simulink library "MIL_Test"  (Simulink 7.0)
values from neighbouring files (symbols this model uses):
  TID = min('TI' == AFT(1:2))    [PAS_callback.m]    (also in PSTID_callback.m = [block '/TID'])
undefined symbols (not defined in the file or in its folder): getdatatypespecs, slcm, StepSize
libraries: simulink x71, MIL_Test x6
(part 6 of 11)

== system MIL_Test/Test Data/Feature generation/Generate timed limited increase/Subsystem/Subsystem39 ==
  In1 : Inport  OutDataType=sfix(16)  OutScaling=2^0
  In2 : Inport  Port=2  OutDataType=sfix(16)  OutScaling=2^0
  In3 : Inport  Port=3  OutDataType=sfix(16)  OutScaling=2^0
  Output1 : Sum  Inputs=|+-+  OutDataType=sfix(16)  OutScaling=2^0  SaturateOnIntegerOverflow=on  InputSameDT=on
  RO : RelationalOperator  Operator=>  LogicOutDataTypeMode=boolean
  Switch : Switch  Criteria=u2 > Threshold
  Out1 : Outport  OutDataType=sfix(16)  OutScaling=2^0
  wires:
  In3/1 -> Output1/3
  Output1/1 -> Switch/1
  RO/1 -> Switch/2
  Switch/1 -> Out1/1
  In2/1 -> RO/1, Output1/1, Switch/3  "U(k)"
  In1/1 -> RO/2, Output1/2

== system MIL_Test/Test Data/Feature generation/Generate timed limited increase/Subsystem/Subsystem4 ==
  In1 : Inport  OutDataType=sfix(16)  OutScaling=2^0
  In2 : Inport  Port=2  OutDataType=sfix(16)  OutScaling=2^0
  In3 : Inport  Port=3  OutDataType=sfix(16)  OutScaling=2^0
  Output1 : Sum  Inputs=|+-+  OutDataType=sfix(16)  OutScaling=2^0  SaturateOnIntegerOverflow=on  InputSameDT=on
  RO : RelationalOperator  Operator=>  LogicOutDataTypeMode=boolean
  Switch : Switch  Criteria=u2 > Threshold
  Out1 : Outport  OutDataType=sfix(16)  OutScaling=2^0
  wires:
  In3/1 -> Output1/3
  Output1/1 -> Switch/1
  RO/1 -> Switch/2
  Switch/1 -> Out1/1
  In2/1 -> RO/1, Output1/1, Switch/3  "U(k)"
  In1/1 -> RO/2, Output1/2

== system MIL_Test/Test Data/Feature generation/Generate timed limited increase/Subsystem/Subsystem40 ==
  In1 : Inport  OutDataType=sfix(16)  OutScaling=2^0
  In2 : Inport  Port=2  OutDataType=sfix(16)  OutScaling=2^0
  In3 : Inport  Port=3  OutDataType=sfix(16)  OutScaling=2^0
  Output1 : Sum  Inputs=|+-+  OutDataType=sfix(16)  OutScaling=2^0  SaturateOnIntegerOverflow=on  InputSameDT=on
  RO : RelationalOperator  Operator=>  LogicOutDataTypeMode=boolean
  Switch : Switch  Criteria=u2 > Threshold
  Out1 : Outport  OutDataType=sfix(16)  OutScaling=2^0
  wires:
  In3/1 -> Output1/3
  Output1/1 -> Switch/1
  RO/1 -> Switch/2
  Switch/1 -> Out1/1
  In2/1 -> RO/1, Output1/1, Switch/3  "U(k)"
  In1/1 -> RO/2, Output1/2

== system MIL_Test/Test Data/Feature generation/Generate timed limited increase/Subsystem/Subsystem41 ==
  In1 : Inport  OutDataType=sfix(16)  OutScaling=2^0
  In2 : Inport  Port=2  OutDataType=sfix(16)  OutScaling=2^0
  In3 : Inport  Port=3  OutDataType=sfix(16)  OutScaling=2^0
  Output1 : Sum  Inputs=|+-+  OutDataType=sfix(16)  OutScaling=2^0  SaturateOnIntegerOverflow=on  InputSameDT=on
  RO : RelationalOperator  Operator=>  LogicOutDataTypeMode=boolean
  Switch : Switch  Criteria=u2 > Threshold
  Out1 : Outport  OutDataType=sfix(16)  OutScaling=2^0
  wires:
  In3/1 -> Output1/3
  Output1/1 -> Switch/1
  RO/1 -> Switch/2
  Switch/1 -> Out1/1
  In2/1 -> RO/1, Output1/1, Switch/3  "U(k)"
  In1/1 -> RO/2, Output1/2

== system MIL_Test/Test Data/Feature generation/Generate timed limited increase/Subsystem/Subsystem42 ==
  In1 : Inport  OutDataType=sfix(16)  OutScaling=2^0
  In2 : Inport  Port=2  OutDataType=sfix(16)  OutScaling=2^0
  In3 : Inport  Port=3  OutDataType=sfix(16)  OutScaling=2^0
  Output1 : Sum  Inputs=|+-+  OutDataType=sfix(16)  OutScaling=2^0  SaturateOnIntegerOverflow=on  InputSameDT=on
  RO : RelationalOperator  Operator=>  LogicOutDataTypeMode=boolean
  Switch : Switch  Criteria=u2 > Threshold
  Out1 : Outport  OutDataType=sfix(16)  OutScaling=2^0
  wires:
  In3/1 -> Output1/3
  Output1/1 -> Switch/1
  RO/1 -> Switch/2
  Switch/1 -> Out1/1
  In2/1 -> RO/1, Output1/1, Switch/3  "U(k)"
  In1/1 -> RO/2, Output1/2

== system MIL_Test/Test Data/Feature generation/Generate timed limited increase/Subsystem/Subsystem43 ==
  In1 : Inport  OutDataType=sfix(16)  OutScaling=2^0
  In2 : Inport  Port=2  OutDataType=sfix(16)  OutScaling=2^0
  In3 : Inport  Port=3  OutDataType=sfix(16)  OutScaling=2^0
  Output1 : Sum  Inputs=|+-+  OutDataType=sfix(16)  OutScaling=2^0  SaturateOnIntegerOverflow=on  InputSameDT=on
  RO : RelationalOperator  Operator=>  LogicOutDataTypeMode=boolean
  Switch : Switch  Criteria=u2 > Threshold
  Out1 : Outport  OutDataType=sfix(16)  OutScaling=2^0
  wires:
  In3/1 -> Output1/3
  Output1/1 -> Switch/1
  RO/1 -> Switch/2
  Switch/1 -> Out1/1
  In2/1 -> RO/1, Output1/1, Switch/3  "U(k)"
  In1/1 -> RO/2, Output1/2

== system MIL_Test/Test Data/Feature generation/Generate timed limited increase/Subsystem/Subsystem44 ==
  In1 : Inport  OutDataType=sfix(16)  OutScaling=2^0
  In2 : Inport  Port=2  OutDataType=sfix(16)  OutScaling=2^0
  In3 : Inport  Port=3  OutDataType=sfix(16)  OutScaling=2^0
  Output1 : Sum  Inputs=|+-+  OutDataType=sfix(16)  OutScaling=2^0  SaturateOnIntegerOverflow=on  InputSameDT=on
  RO : RelationalOperator  Operator=>  LogicOutDataTypeMode=boolean
  Switch : Switch  Criteria=u2 > Threshold
  Out1 : Outport  OutDataType=sfix(16)  OutScaling=2^0
  wires:
  In3/1 -> Output1/3
  Output1/1 -> Switch/1
  RO/1 -> Switch/2
  Switch/1 -> Out1/1
  In2/1 -> RO/1, Output1/1, Switch/3  "U(k)"
  In1/1 -> RO/2, Output1/2

== system MIL_Test/Test Data/Feature generation/Generate timed limited increase/Subsystem/Subsystem45 ==
  In1 : Inport  OutDataType=sfix(16)  OutScaling=2^0
  In2 : Inport  Port=2  OutDataType=sfix(16)  OutScaling=2^0
  In3 : Inport  Port=3  OutDataType=sfix(16)  OutScaling=2^0
  Output1 : Sum  Inputs=|+-+  OutDataType=sfix(16)  OutScaling=2^0  SaturateOnIntegerOverflow=on  InputSameDT=on
  RO : RelationalOperator  Operator=>  LogicOutDataTypeMode=boolean
  Switch : Switch  Criteria=u2 > Threshold
  Out1 : Outport  OutDataType=sfix(16)  OutScaling=2^0
  wires:
  In3/1 -> Output1/3
  Output1/1 -> Switch/1
  RO/1 -> Switch/2
  Switch/1 -> Out1/1
  In2/1 -> RO/1, Output1/1, Switch/3  "U(k)"
  In1/1 -> RO/2, Output1/2

== system MIL_Test/Test Data/Feature generation/Generate timed limited increase/Subsystem/Subsystem46 ==
  In1 : Inport  OutDataType=sfix(16)  OutScaling=2^0
  In2 : Inport  Port=2  OutDataType=sfix(16)  OutScaling=2^0
  In3 : Inport  Port=3  OutDataType=sfix(16)  OutScaling=2^0
  Output1 : Sum  Inputs=|+-+  OutDataType=sfix(16)  OutScaling=2^0  SaturateOnIntegerOverflow=on  InputSameDT=on
  RO : RelationalOperator  Operator=>  LogicOutDataTypeMode=boolean
  Switch : Switch  Criteria=u2 > Threshold
  Out1 : Outport  OutDataType=sfix(16)  OutScaling=2^0
  wires:
  In3/1 -> Output1/3
  Output1/1 -> Switch/1
  RO/1 -> Switch/2
  Switch/1 -> Out1/1
  In2/1 -> RO/1, Output1/1, Switch/3  "U(k)"
  In1/1 -> RO/2, Output1/2

== system MIL_Test/Test Data/Feature generation/Generate timed limited increase/Subsystem/Subsystem47 ==
  In1 : Inport  OutDataType=sfix(16)  OutScaling=2^0
  In2 : Inport  Port=2  OutDataType=sfix(16)  OutScaling=2^0
  In3 : Inport  Port=3  OutDataType=sfix(16)  OutScaling=2^0
  Output1 : Sum  Inputs=|+-+  OutDataType=sfix(16)  OutScaling=2^0  SaturateOnIntegerOverflow=on  InputSameDT=on
  RO : RelationalOperator  Operator=>  LogicOutDataTypeMode=boolean
  Switch : Switch  Criteria=u2 > Threshold
  Out1 : Outport  OutDataType=sfix(16)  OutScaling=2^0
  wires:
  In3/1 -> Output1/3
  Output1/1 -> Switch/1
  RO/1 -> Switch/2
  Switch/1 -> Out1/1
  In2/1 -> RO/1, Output1/1, Switch/3  "U(k)"
  In1/1 -> RO/2, Output1/2

== system MIL_Test/Test Data/Feature generation/Generate timed limited increase/Subsystem/Subsystem48 ==
  In1 : Inport  OutDataType=sfix(16)  OutScaling=2^0
  In2 : Inport  Port=2  OutDataType=sfix(16)  OutScaling=2^0
  In3 : Inport  Port=3  OutDataType=sfix(16)  OutScaling=2^0
  Output1 : Sum  Inputs=|+-+  OutDataType=sfix(16)  OutScaling=2^0  SaturateOnIntegerOverflow=on  InputSameDT=on
  RO : RelationalOperator  Operator=>  LogicOutDataTypeMode=boolean
  Switch : Switch  Criteria=u2 > Threshold
  Out1 : Outport  OutDataType=sfix(16)  OutScaling=2^0
  wires:
  In3/1 -> Output1/3
  Output1/1 -> Switch/1
  RO/1 -> Switch/2
  Switch/1 -> Out1/1
  In2/1 -> RO/1, Output1/1, Switch/3  "U(k)"
  In1/1 -> RO/2, Output1/2

== system MIL_Test/Test Data/Feature generation/Generate timed limited increase/Subsystem/Subsystem49 ==
  In1 : Inport  OutDataType=sfix(16)  OutScaling=2^0
  In2 : Inport  Port=2  OutDataType=sfix(16)  OutScaling=2^0
  In3 : Inport  Port=3  OutDataType=sfix(16)  OutScaling=2^0
  Output1 : Sum  Inputs=|+-+  OutDataType=sfix(16)  OutScaling=2^0  SaturateOnIntegerOverflow=on  InputSameDT=on
  RO : RelationalOperator  Operator=>  LogicOutDataTypeMode=boolean
  Switch : Switch  Criteria=u2 > Threshold
  Out1 : Outport  OutDataType=sfix(16)  OutScaling=2^0
  wires:
  In3/1 -> Output1/3
  Output1/1 -> Switch/1
  RO/1 -> Switch/2
  Switch/1 -> Out1/1
  In2/1 -> RO/1, Output1/1, Switch/3  "U(k)"
  In1/1 -> RO/2, Output1/2

== system MIL_Test/Test Data/Feature generation/Generate timed limited increase/Subsystem/Subsystem5 ==
  In1 : Inport  OutDataType=sfix(16)  OutScaling=2^0
  In2 : Inport  Port=2  OutDataType=sfix(16)  OutScaling=2^0
  In3 : Inport  Port=3  OutDataType=sfix(16)  OutScaling=2^0
  Output1 : Sum  Inputs=|+-+  OutDataType=sfix(16)  OutScaling=2^0  SaturateOnIntegerOverflow=on  InputSameDT=on
  RO : RelationalOperator  Operator=>  LogicOutDataTypeMode=boolean
  Switch : Switch  Criteria=u2 > Threshold
  Out1 : Outport  OutDataType=sfix(16)  OutScaling=2^0
  wires:
  In3/1 -> Output1/3
  Output1/1 -> Switch/1
  RO/1 -> Switch/2
  Switch/1 -> Out1/1
  In2/1 -> RO/1, Output1/1, Switch/3  "U(k)"
  In1/1 -> RO/2, Output1/2

== system MIL_Test/Test Data/Feature generation/Generate timed limited increase/Subsystem/Subsystem50 ==
  In1 : Inport  OutDataType=sfix(16)  OutScaling=2^0
  In2 : Inport  Port=2  OutDataType=sfix(16)  OutScaling=2^0
  In3 : Inport  Port=3  OutDataType=sfix(16)  OutScaling=2^0
  Output1 : Sum  Inputs=|+-+  OutDataType=sfix(16)  OutScaling=2^0  SaturateOnIntegerOverflow=on  InputSameDT=on
  RO : RelationalOperator  Operator=>  LogicOutDataTypeMode=boolean
  Switch : Switch  Criteria=u2 > Threshold
  Out1 : Outport  OutDataType=sfix(16)  OutScaling=2^0
  wires:
  In3/1 -> Output1/3
  Output1/1 -> Switch/1
  RO/1 -> Switch/2
  Switch/1 -> Out1/1
  In2/1 -> RO/1, Output1/1, Switch/3  "U(k)"
  In1/1 -> RO/2, Output1/2

== system MIL_Test/Test Data/Feature generation/Generate timed limited increase/Subsystem/Subsystem51 ==
  In1 : Inport  OutDataType=sfix(16)  OutScaling=2^0
  In2 : Inport  Port=2  OutDataType=sfix(16)  OutScaling=2^0
  In3 : Inport  Port=3  OutDataType=sfix(16)  OutScaling=2^0
  Output1 : Sum  Inputs=|+-+  OutDataType=sfix(16)  OutScaling=2^0  SaturateOnIntegerOverflow=on  InputSameDT=on
  RO : RelationalOperator  Operator=>  LogicOutDataTypeMode=boolean
  Switch : Switch  Criteria=u2 > Threshold
  Out1 : Outport  OutDataType=sfix(16)  OutScaling=2^0
  wires:
  In3/1 -> Output1/3
  Output1/1 -> Switch/1
  RO/1 -> Switch/2
  Switch/1 -> Out1/1
  In2/1 -> RO/1, Output1/1, Switch/3  "U(k)"
  In1/1 -> RO/2, Output1/2

== system MIL_Test/Test Data/Feature generation/Generate timed limited increase/Subsystem/Subsystem52 ==
  In1 : Inport  OutDataType=sfix(16)  OutScaling=2^0
  In2 : Inport  Port=2  OutDataType=sfix(16)  OutScaling=2^0
  In3 : Inport  Port=3  OutDataType=sfix(16)  OutScaling=2^0
  Output1 : Sum  Inputs=|+-+  OutDataType=sfix(16)  OutScaling=2^0  SaturateOnIntegerOverflow=on  InputSameDT=on
  RO : RelationalOperator  Operator=>  LogicOutDataTypeMode=boolean
  Switch : Switch  Criteria=u2 > Threshold
  Out1 : Outport  OutDataType=sfix(16)  OutScaling=2^0
  wires:
  In3/1 -> Output1/3
  Output1/1 -> Switch/1
  RO/1 -> Switch/2
  Switch/1 -> Out1/1
  In2/1 -> RO/1, Output1/1, Switch/3  "U(k)"
  In1/1 -> RO/2, Output1/2

== system MIL_Test/Test Data/Feature generation/Generate timed limited increase/Subsystem/Subsystem53 ==
  In1 : Inport  OutDataType=sfix(16)  OutScaling=2^0
  In2 : Inport  Port=2  OutDataType=sfix(16)  OutScaling=2^0
  In3 : Inport  Port=3  OutDataType=sfix(16)  OutScaling=2^0
  Output1 : Sum  Inputs=|+-+  OutDataType=sfix(16)  OutScaling=2^0  SaturateOnIntegerOverflow=on  InputSameDT=on
  RO : RelationalOperator  Operator=>  LogicOutDataTypeMode=boolean
  Switch : Switch  Criteria=u2 > Threshold
  Out1 : Outport  OutDataType=sfix(16)  OutScaling=2^0
  wires:
  In3/1 -> Output1/3
  Output1/1 -> Switch/1
  RO/1 -> Switch/2
  Switch/1 -> Out1/1
  In2/1 -> RO/1, Output1/1, Switch/3  "U(k)"
  In1/1 -> RO/2, Output1/2

== system MIL_Test/Test Data/Feature generation/Generate timed limited increase/Subsystem/Subsystem54 ==
  In1 : Inport  OutDataType=sfix(16)  OutScaling=2^0
  In2 : Inport  Port=2  OutDataType=sfix(16)  OutScaling=2^0
  In3 : Inport  Port=3  OutDataType=sfix(16)  OutScaling=2^0
  Output1 : Sum  Inputs=|+-+  OutDataType=sfix(16)  OutScaling=2^0  SaturateOnIntegerOverflow=on  InputSameDT=on
  RO : RelationalOperator  Operator=>  LogicOutDataTypeMode=boolean
  Switch : Switch  Criteria=u2 > Threshold
  Out1 : Outport  OutDataType=sfix(16)  OutScaling=2^0
  wires:
  In3/1 -> Output1/3
  Output1/1 -> Switch/1
  RO/1 -> Switch/2
  Switch/1 -> Out1/1
  In2/1 -> RO/1, Output1/1, Switch/3  "U(k)"
  In1/1 -> RO/2, Output1/2

== system MIL_Test/Test Data/Feature generation/Generate timed limited increase/Subsystem/Subsystem55 ==
  In1 : Inport  OutDataType=sfix(16)  OutScaling=2^0
  In2 : Inport  Port=2  OutDataType=sfix(16)  OutScaling=2^0
  In3 : Inport  Port=3  OutDataType=sfix(16)  OutScaling=2^0
  Output1 : Sum  Inputs=|+-+  OutDataType=sfix(16)  OutScaling=2^0  SaturateOnIntegerOverflow=on  InputSameDT=on
  RO : RelationalOperator  Operator=>  LogicOutDataTypeMode=boolean
  Switch : Switch  Criteria=u2 > Threshold
  Out1 : Outport  OutDataType=sfix(16)  OutScaling=2^0
  wires:
  In3/1 -> Output1/3
  Output1/1 -> Switch/1
  RO/1 -> Switch/2
  Switch/1 -> Out1/1
  In2/1 -> RO/1, Output1/1, Switch/3  "U(k)"
  In1/1 -> RO/2, Output1/2

== system MIL_Test/Test Data/Feature generation/Generate timed limited increase/Subsystem/Subsystem56 ==
  In1 : Inport  OutDataType=sfix(16)  OutScaling=2^0
  In2 : Inport  Port=2  OutDataType=sfix(16)  OutScaling=2^0
  In3 : Inport  Port=3  OutDataType=sfix(16)  OutScaling=2^0
  Output1 : Sum  Inputs=|+-+  OutDataType=sfix(16)  OutScaling=2^0  SaturateOnIntegerOverflow=on  InputSameDT=on
  RO : RelationalOperator  Operator=>  LogicOutDataTypeMode=boolean
  Switch : Switch  Criteria=u2 > Threshold
  Out1 : Outport  OutDataType=sfix(16)  OutScaling=2^0
  wires:
  In3/1 -> Output1/3
  Output1/1 -> Switch/1
  RO/1 -> Switch/2
  Switch/1 -> Out1/1
  In2/1 -> RO/1, Output1/1, Switch/3  "U(k)"
  In1/1 -> RO/2, Output1/2

== system MIL_Test/Test Data/Feature generation/Generate timed limited increase/Subsystem/Subsystem57 ==
  In1 : Inport  OutDataType=sfix(16)  OutScaling=2^0
  In2 : Inport  Port=2  OutDataType=sfix(16)  OutScaling=2^0
  In3 : Inport  Port=3  OutDataType=sfix(16)  OutScaling=2^0
  Output1 : Sum  Inputs=|+-+  OutDataType=sfix(16)  OutScaling=2^0  SaturateOnIntegerOverflow=on  InputSameDT=on
  RO : RelationalOperator  Operator=>  LogicOutDataTypeMode=boolean
  Switch : Switch  Criteria=u2 > Threshold
  Out1 : Outport  OutDataType=sfix(16)  OutScaling=2^0
  wires:
  In3/1 -> Output1/3
  Output1/1 -> Switch/1
  RO/1 -> Switch/2
  Switch/1 -> Out1/1
  In2/1 -> RO/1, Output1/1, Switch/3  "U(k)"
  In1/1 -> RO/2, Output1/2

== system MIL_Test/Test Data/Feature generation/Generate timed limited increase/Subsystem/Subsystem58 ==
  In1 : Inport  OutDataType=sfix(16)  OutScaling=2^0
  In2 : Inport  Port=2  OutDataType=sfix(16)  OutScaling=2^0
  In3 : Inport  Port=3  OutDataType=sfix(16)  OutScaling=2^0
  Output1 : Sum  Inputs=|+-+  OutDataType=sfix(16)  OutScaling=2^0  SaturateOnIntegerOverflow=on  InputSameDT=on
  RO : RelationalOperator  Operator=>  LogicOutDataTypeMode=boolean
  Switch : Switch  Criteria=u2 > Threshold
  Out1 : Outport  OutDataType=sfix(16)  OutScaling=2^0
  wires:
  In3/1 -> Output1/3
  Output1/1 -> Switch/1
  RO/1 -> Switch/2
  Switch/1 -> Out1/1
  In2/1 -> RO/1, Output1/1, Switch/3  "U(k)"
  In1/1 -> RO/2, Output1/2

== system MIL_Test/Test Data/Feature generation/Generate timed limited increase/Subsystem/Subsystem59 ==
  In1 : Inport  OutDataType=sfix(16)  OutScaling=2^0
  In2 : Inport  Port=2  OutDataType=sfix(16)  OutScaling=2^0
  In3 : Inport  Port=3  OutDataType=sfix(16)  OutScaling=2^0
  Output1 : Sum  Inputs=|+-+  OutDataType=sfix(16)  OutScaling=2^0  SaturateOnIntegerOverflow=on  InputSameDT=on
  RO : RelationalOperator  Operator=>  LogicOutDataTypeMode=boolean
  Switch : Switch  Criteria=u2 > Threshold
  Out1 : Outport  OutDataType=sfix(16)  OutScaling=2^0
  wires:
  In3/1 -> Output1/3
  Output1/1 -> Switch/1
  RO/1 -> Switch/2
  Switch/1 -> Out1/1
  In2/1 -> RO/1, Output1/1, Switch/3  "U(k)"
  In1/1 -> RO/2, Output1/2

== system MIL_Test/Test Data/Feature generation/Generate timed limited increase/Subsystem/Subsystem6 ==
  In1 : Inport  OutDataType=sfix(16)  OutScaling=2^0
  In2 : Inport  Port=2  OutDataType=sfix(16)  OutScaling=2^0
  In3 : Inport  Port=3  OutDataType=sfix(16)  OutScaling=2^0
  Output1 : Sum  Inputs=|+-+  OutDataType=sfix(16)  OutScaling=2^0  SaturateOnIntegerOverflow=on  InputSameDT=on
  RO : RelationalOperator  Operator=>  LogicOutDataTypeMode=boolean
  Switch : Switch  Criteria=u2 > Threshold
  Out1 : Outport  OutDataType=sfix(16)  OutScaling=2^0
  wires:
  In3/1 -> Output1/3
  Output1/1 -> Switch/1
  RO/1 -> Switch/2
  Switch/1 -> Out1/1
  In2/1 -> RO/1, Output1/1, Switch/3  "U(k)"
  In1/1 -> RO/2, Output1/2

== system MIL_Test/Test Data/Feature generation/Generate timed limited increase/Subsystem/Subsystem60 ==
  In1 : Inport  OutDataType=sfix(16)  OutScaling=2^0
  In2 : Inport  Port=2  OutDataType=sfix(16)  OutScaling=2^0
  In3 : Inport  Port=3  OutDataType=sfix(16)  OutScaling=2^0
  Output1 : Sum  Inputs=|+-+  OutDataType=sfix(16)  OutScaling=2^0  SaturateOnIntegerOverflow=on  InputSameDT=on
  RO : RelationalOperator  Operator=>  LogicOutDataTypeMode=boolean
  Switch : Switch  Criteria=u2 > Threshold
  Out1 : Outport  OutDataType=sfix(16)  OutScaling=2^0
  wires:
  In3/1 -> Output1/3
  Output1/1 -> Switch/1
  RO/1 -> Switch/2
  Switch/1 -> Out1/1
  In2/1 -> RO/1, Output1/1, Switch/3  "U(k)"
  In1/1 -> RO/2, Output1/2

== system MIL_Test/Test Data/Feature generation/Generate timed limited increase/Subsystem/Subsystem61 ==
  In1 : Inport  OutDataType=sfix(16)  OutScaling=2^0
  In2 : Inport  Port=2  OutDataType=sfix(16)  OutScaling=2^0
  In3 : Inport  Port=3  OutDataType=sfix(16)  OutScaling=2^0
  Output1 : Sum  Inputs=|+-+  OutDataType=sfix(16)  OutScaling=2^0  SaturateOnIntegerOverflow=on  InputSameDT=on
  RO : RelationalOperator  Operator=>  LogicOutDataTypeMode=boolean
  Switch : Switch  Criteria=u2 > Threshold
  Out1 : Outport  OutDataType=sfix(16)  OutScaling=2^0
  wires:
  In3/1 -> Output1/3
  Output1/1 -> Switch/1
  RO/1 -> Switch/2
  Switch/1 -> Out1/1
  In2/1 -> RO/1, Output1/1, Switch/3  "U(k)"
  In1/1 -> RO/2, Output1/2

== system MIL_Test/Test Data/Feature generation/Generate timed limited increase/Subsystem/Subsystem62 ==
  In1 : Inport  OutDataType=sfix(16)  OutScaling=2^0
  In2 : Inport  Port=2  OutDataType=sfix(16)  OutScaling=2^0
  In3 : Inport  Port=3  OutDataType=sfix(16)  OutScaling=2^0
  Output1 : Sum  Inputs=|+-+  OutDataType=sfix(16)  OutScaling=2^0  SaturateOnIntegerOverflow=on  InputSameDT=on
  RO : RelationalOperator  Operator=>  LogicOutDataTypeMode=boolean
  Switch : Switch  Criteria=u2 > Threshold
  Out1 : Outport  OutDataType=sfix(16)  OutScaling=2^0
  wires:
  In3/1 -> Output1/3
  Output1/1 -> Switch/1
  RO/1 -> Switch/2
  Switch/1 -> Out1/1
  In2/1 -> RO/1, Output1/1, Switch/3  "U(k)"
  In1/1 -> RO/2, Output1/2

== system MIL_Test/Test Data/Feature generation/Generate timed limited increase/Subsystem/Subsystem63 ==
  In1 : Inport  OutDataType=sfix(16)  OutScaling=2^0
  In2 : Inport  Port=2  OutDataType=sfix(16)  OutScaling=2^0
  In3 : Inport  Port=3  OutDataType=sfix(16)  OutScaling=2^0
  Output1 : Sum  Inputs=|+-+  OutDataType=sfix(16)  OutScaling=2^0  SaturateOnIntegerOverflow=on  InputSameDT=on
  RO : RelationalOperator  Operator=>  LogicOutDataTypeMode=boolean
  Switch : Switch  Criteria=u2 > Threshold
  Out1 : Outport  OutDataType=sfix(16)  OutScaling=2^0
  wires:
  In3/1 -> Output1/3
  Output1/1 -> Switch/1
  RO/1 -> Switch/2
  Switch/1 -> Out1/1
  In2/1 -> RO/1, Output1/1, Switch/3  "U(k)"
  In1/1 -> RO/2, Output1/2

== system MIL_Test/Test Data/Feature generation/Generate timed limited increase/Subsystem/Subsystem64 ==
  In1 : Inport  OutDataType=sfix(16)  OutScaling=2^0
  In2 : Inport  Port=2  OutDataType=sfix(16)  OutScaling=2^0
  In3 : Inport  Port=3  OutDataType=sfix(16)  OutScaling=2^0
  Output1 : Sum  Inputs=|+-+  OutDataType=sfix(16)  OutScaling=2^0  SaturateOnIntegerOverflow=on  InputSameDT=on
  RO : RelationalOperator  Operator=>  LogicOutDataTypeMode=boolean
  Switch : Switch  Criteria=u2 > Threshold
  Out1 : Outport  OutDataType=sfix(16)  OutScaling=2^0
  wires:
  In3/1 -> Output1/3
  Output1/1 -> Switch/1
  RO/1 -> Switch/2
  Switch/1 -> Out1/1
  In2/1 -> RO/1, Output1/1, Switch/3  "U(k)"
  In1/1 -> RO/2, Output1/2

== system MIL_Test/Test Data/Feature generation/Generate timed limited increase/Subsystem/Subsystem65 ==
  In1 : Inport  OutDataType=sfix(16)  OutScaling=2^0
  In2 : Inport  Port=2  OutDataType=sfix(16)  OutScaling=2^0
  In3 : Inport  Port=3  OutDataType=sfix(16)  OutScaling=2^0
  Output1 : Sum  Inputs=|+-+  OutDataType=sfix(16)  OutScaling=2^0  SaturateOnIntegerOverflow=on  InputSameDT=on
  RO : RelationalOperator  Operator=>  LogicOutDataTypeMode=boolean
  Switch : Switch  Criteria=u2 > Threshold
  Out1 : Outport  OutDataType=sfix(16)  OutScaling=2^0
  wires:
  In3/1 -> Output1/3
  Output1/1 -> Switch/1
  RO/1 -> Switch/2
  Switch/1 -> Out1/1
  In2/1 -> RO/1, Output1/1, Switch/3  "U(k)"
  In1/1 -> RO/2, Output1/2

== system MIL_Test/Test Data/Feature generation/Generate timed limited increase/Subsystem/Subsystem66 ==
  In1 : Inport  OutDataType=sfix(16)  OutScaling=2^0
  In2 : Inport  Port=2  OutDataType=sfix(16)  OutScaling=2^0
  In3 : Inport  Port=3  OutDataType=sfix(16)  OutScaling=2^0
  Output1 : Sum  Inputs=|+-+  OutDataType=sfix(16)  OutScaling=2^0  SaturateOnIntegerOverflow=on  InputSameDT=on
  RO : RelationalOperator  Operator=>  LogicOutDataTypeMode=boolean
  Switch : Switch  Criteria=u2 > Threshold
  Out1 : Outport  OutDataType=sfix(16)  OutScaling=2^0
  wires:
  In3/1 -> Output1/3
  Output1/1 -> Switch/1
  RO/1 -> Switch/2
  Switch/1 -> Out1/1
  In2/1 -> RO/1, Output1/1, Switch/3  "U(k)"
  In1/1 -> RO/2, Output1/2

== system MIL_Test/Test Data/Feature generation/Generate timed limited increase/Subsystem/Subsystem67 ==
  In1 : Inport  OutDataType=sfix(16)  OutScaling=2^0
  In2 : Inport  Port=2  OutDataType=sfix(16)  OutScaling=2^0
  In3 : Inport  Port=3  OutDataType=sfix(16)  OutScaling=2^0
  Output1 : Sum  Inputs=|+-+  OutDataType=sfix(16)  OutScaling=2^0  SaturateOnIntegerOverflow=on  InputSameDT=on
  RO : RelationalOperator  Operator=>  LogicOutDataTypeMode=boolean
  Switch : Switch  Criteria=u2 > Threshold
  Out1 : Outport  OutDataType=sfix(16)  OutScaling=2^0
  wires:
  In3/1 -> Output1/3
  Output1/1 -> Switch/1
  RO/1 -> Switch/2
  Switch/1 -> Out1/1
  In2/1 -> RO/1, Output1/1, Switch/3  "U(k)"
  In1/1 -> RO/2, Output1/2

== system MIL_Test/Test Data/Feature generation/Generate timed limited increase/Subsystem/Subsystem68 ==
  In1 : Inport  OutDataType=sfix(16)  OutScaling=2^0
  In2 : Inport  Port=2  OutDataType=sfix(16)  OutScaling=2^0
  In3 : Inport  Port=3  OutDataType=sfix(16)  OutScaling=2^0
  Output1 : Sum  Inputs=|+-+  OutDataType=sfix(16)  OutScaling=2^0  SaturateOnIntegerOverflow=on  InputSameDT=on
  RO : RelationalOperator  Operator=>  LogicOutDataTypeMode=boolean
  Switch : Switch  Criteria=u2 > Threshold
  Out1 : Outport  OutDataType=sfix(16)  OutScaling=2^0
  wires:
  In3/1 -> Output1/3
  Output1/1 -> Switch/1
  RO/1 -> Switch/2
  Switch/1 -> Out1/1
  In2/1 -> RO/1, Output1/1, Switch/3  "U(k)"
  In1/1 -> RO/2, Output1/2

== system MIL_Test/Test Data/Feature generation/Generate timed limited increase/Subsystem/Subsystem69 ==
  In1 : Inport  OutDataType=sfix(16)  OutScaling=2^0
  In2 : Inport  Port=2  OutDataType=sfix(16)  OutScaling=2^0
  In3 : Inport  Port=3  OutDataType=sfix(16)  OutScaling=2^0
  Output1 : Sum  Inputs=|+-+  OutDataType=sfix(16)  OutScaling=2^0  SaturateOnIntegerOverflow=on  InputSameDT=on
  RO : RelationalOperator  Operator=>  LogicOutDataTypeMode=boolean
  Switch : Switch  Criteria=u2 > Threshold
  Out1 : Outport  OutDataType=sfix(16)  OutScaling=2^0
  wires:
  In3/1 -> Output1/3
  Output1/1 -> Switch/1
  RO/1 -> Switch/2
  Switch/1 -> Out1/1
  In2/1 -> RO/1, Output1/1, Switch/3  "U(k)"
  In1/1 -> RO/2, Output1/2

== system MIL_Test/Test Data/Feature generation/Generate timed limited increase/Subsystem/Subsystem7 ==
  In1 : Inport  OutDataType=sfix(16)  OutScaling=2^0
  In2 : Inport  Port=2  OutDataType=sfix(16)  OutScaling=2^0
  In3 : Inport  Port=3  OutDataType=sfix(16)  OutScaling=2^0
  Output1 : Sum  Inputs=|+-+  OutDataType=sfix(16)  OutScaling=2^0  SaturateOnIntegerOverflow=on  InputSameDT=on
  RO : RelationalOperator  Operator=>  LogicOutDataTypeMode=boolean
  Switch : Switch  Criteria=u2 > Threshold
  Out1 : Outport  OutDataType=sfix(16)  OutScaling=2^0
  wires:
  In3/1 -> Output1/3
  Output1/1 -> Switch/1
  RO/1 -> Switch/2
  Switch/1 -> Out1/1
  In2/1 -> RO/1, Output1/1, Switch/3  "U(k)"
  In1/1 -> RO/2, Output1/2

== system MIL_Test/Test Data/Feature generation/Generate timed limited increase/Subsystem/Subsystem70 ==
  In1 : Inport  OutDataType=sfix(16)  OutScaling=2^0
  In2 : Inport  Port=2  OutDataType=sfix(16)  OutScaling=2^0
  In3 : Inport  Port=3  OutDataType=sfix(16)  OutScaling=2^0
  Output1 : Sum  Inputs=|+-+  OutDataType=sfix(16)  OutScaling=2^0  SaturateOnIntegerOverflow=on  InputSameDT=on
  RO : RelationalOperator  Operator=>  LogicOutDataTypeMode=boolean
  Switch : Switch  Criteria=u2 > Threshold
  Out1 : Outport  OutDataType=sfix(16)  OutScaling=2^0
  wires:
  In3/1 -> Output1/3
  Output1/1 -> Switch/1
  RO/1 -> Switch/2
  Switch/1 -> Out1/1
  In2/1 -> RO/1, Output1/1, Switch/3  "U(k)"
  In1/1 -> RO/2, Output1/2

== system MIL_Test/Test Data/Feature generation/Generate timed limited increase/Subsystem/Subsystem8 ==
  In1 : Inport  OutDataType=sfix(16)  OutScaling=2^0
  In2 : Inport  Port=2  OutDataType=sfix(16)  OutScaling=2^0
  In3 : Inport  Port=3  OutDataType=sfix(16)  OutScaling=2^0
  Output1 : Sum  Inputs=|+-+  OutDataType=sfix(16)  OutScaling=2^0  SaturateOnIntegerOverflow=on  InputSameDT=on
  RO : RelationalOperator  Operator=>  LogicOutDataTypeMode=boolean
  Switch : Switch  Criteria=u2 > Threshold
  Out1 : Outport  OutDataType=sfix(16)  OutScaling=2^0
  wires:
  In3/1 -> Output1/3
  Output1/1 -> Switch/1
  RO/1 -> Switch/2
  Switch/1 -> Out1/1
  In2/1 -> RO/1, Output1/1, Switch/3  "U(k)"
  In1/1 -> RO/2, Output1/2

== system MIL_Test/Test Data/Feature generation/Generate timed limited increase/Subsystem/Subsystem9 ==
  In1 : Inport  OutDataType=sfix(16)  OutScaling=2^0
  In2 : Inport  Port=2  OutDataType=sfix(16)  OutScaling=2^0
  In3 : Inport  Port=3  OutDataType=sfix(16)  OutScaling=2^0
  Output1 : Sum  Inputs=|+-+  OutDataType=sfix(16)  OutScaling=2^0  SaturateOnIntegerOverflow=on  InputSameDT=on
  RO : RelationalOperator  Operator=>  LogicOutDataTypeMode=boolean
  Switch : Switch  Criteria=u2 > Threshold
  Out1 : Outport  OutDataType=sfix(16)  OutScaling=2^0
  wires:
  In3/1 -> Output1/3
  Output1/1 -> Switch/1
  RO/1 -> Switch/2
  Switch/1 -> Out1/1
  In2/1 -> RO/1, Output1/1, Switch/3  "U(k)"
  In1/1 -> RO/2, Output1/2

== system MIL_Test/Test Data/Test Data Architecture/<Test data generator>/<Requirement name>/<Preconditions name> ==
  Out Bus : Inport  OutDataType=sfix(16)  OutScaling=2^0
  <Check> : Subsystem
  Feature generation : Subsystem  TreatAsAtomicUnit=on  mask{Param=0}
      mask prompts: Param "Mask Parameter 1:"
  Activate : Outport  OutDataType=sfix(16)  OutScaling=2^0
  <signal1> : Outport  Port=2  OutDataType=sfix(16)  OutScaling=2^0
  wires:
  <Check>/1(A) -> Activate/1
  Feature generation/1(<signal1>) -> <signal1>/1
  Out Bus/1 -> <Check>/1(Out Bus)

== system MIL_Test/Test Data/Test Data Architecture/<Test data generator>/<Requirement name>/Initialisation & Stabilisation ==
  <Feature generation> : Subsystem  TreatAsAtomicUnit=on  mask{Param=0}
      mask prompts: Param "Mask Parameter 1:"
  <signal1> : Outport  OutDataType=sfix(16)  OutScaling=2^0
  wires:
  <Feature generation>/1(<signal1>) -> <signal1>/1

== system MIL_Test/Validation Function/Feature extraction/Complete step detection/Step detection/Active if signals constant for some specified time ==
  Signal1 : Inport  OutDataType=sfix(16)  OutScaling=2^0
  Signal 2 : Inport  Port=2  OutDataType=sfix(16)  OutScaling=2^0
  Logical Operator1 : Logic  AllPortsSameDT=off  OutDataTypeMode=boolean
  Min Time : Constant  Value=10  OutDataType=sfix(16)  OutScaling=2^0
  MinMax : MinMax  Inputs=2  OutDataType=sfix(16)  OutScaling=2^0
  Relational Operator2 : RelationalOperator  Operator=<=  LogicOutDataTypeMode=boolean
  Switch : Switch  Criteria=u2 ~= 0
  Time since signal constant : Subsystem  TreatAsAtomicUnit=on  mask(Feature extraction block){RT=0.001}
      mask prompts: RT "Relative tolerance in %"
      mask help: Detect if the signal value is constant (using the last two signal values) allowing for a user-defined relative deviation
      mask CallbackString:
      | if or( (str2double(get_param(gcb,'RT')) < 0), (str2double(get_param(gcb,'RT')) > 100))
      |     error(['Relative tolerance value (' get_param(gcb,'RT') ') out of range. Please give a value between 0 and 100.']);
      | else
      |     set_param([gcb '/Detect constant/Relative tolerance/Relative Tolerance'],'Value',get_param(gcb,'RT'));
      |     set_param([gcb '/Detect constant'],'RT',get_param(gcb,'RT'));
      | end
  Time since signal constant1 : Subsystem  TreatAsAtomicUnit=on  mask(Feature extraction block){RT=0.001}
      mask prompts: RT "Relative tolerance in %"
      mask help: Detect if the signal value is constant (using the last two signal values) allowing for a user-defined relative deviation
      mask CallbackString:
      | if or( (str2double(get_param(gcb,'RT')) < 0), (str2double(get_param(gcb,'RT')) > 100))
      |     error(['Relative tolerance value (' get_param(gcb,'RT') ') out of range. Please give a value between 0 and 100.']);
      | else
      |     set_param([gcb '/Detect constant/Relative tolerance/Relative Tolerance'],'Value',get_param(gcb,'RT'));
      |     set_param([gcb '/Detect constant'],'RT',get_param(gcb,'RT'));
      | end
  Zero : Constant  Value=0  OutDataType=sfix(16)  OutScaling=2^0
  Constant signals : Outport  OutDataType=sfix(16)  OutScaling=2^0
  wires:
  Zero/1 -> Switch/3
  Logical Operator1/1 -> Switch/2
  MinMax/1 -> Switch/1
  Time since signal constant1/1(Trigger) -> Logical Operator1/2
  Time since signal constant/1(Trigger) -> Logical Operator1/1
  Time since signal constant/2(Feature) -> MinMax/1
  Time since signal constant1/2(Feature) -> MinMax/2
  Switch/1 -> Relational Operator2/2
  Min Time/1 -> Relational Operator2/1
  Relational Operator2/1 -> Constant signals/1
  Signal 2/1 -> Time since signal constant1/1(Signal)
  Signal1/1 -> Time since signal constant/1(Signal)

== system MIL_Test/Validation Function/Feature extraction/Complete step detection/Step detection/Detect constant ==
  Signal : Inport  OutDataType=sfix(16)  OutScaling=2^0
  Clock : Clock
      settings: Decimation=10
  Constant1 : Constant  Value=0  OutDataTypeMode=boolean  OutDataType=sfix(16)  OutScaling=2^0
  Memory : Memory
  Relative tolerance : Subsystem
  Switch : Switch  Criteria=u2 > Threshold
  Constant : Outport  OutDataType=sfix(16)  OutScaling=2^0
  wires:
  Signal/1 -> Memory/1, Relative tolerance/1(sig)
  Memory/1 -> Relative tolerance/2(ref)
  Constant1/1 -> Switch/3
  Clock/1 -> Switch/2
  Relative tolerance/1(sig == ref) -> Switch/1
  Switch/1 -> Constant/1

== system MIL_Test/Validation Function/Feature extraction/Complete step detection/Step detection/Detect decrease ==
  Signal : Inport  OutDataType=sfix(16)  OutScaling=2^0
  Clock : Clock
      settings: Decimation=10
  Memory : Memory
  Relational Operator : RelationalOperator  Operator=<  LogicOutDataTypeMode=Specify via dialog
  Switch : Switch  Criteria=u2 > Threshold
  Decrease : Outport  OutDataType=sfix(16)  OutScaling=2^0
  wires:
  Signal/1 -> Relational Operator/1, Memory/1, Switch/3
  Relational Operator/1 -> Decrease/1
  Clock/1 -> Switch/2
  Memory/1 -> Switch/1
  Switch/1 -> Relational Operator/2

== system MIL_Test/Validation Function/Feature extraction/Complete step detection/Step detection/Detect increase ==
  Signal : Inport  OutDataType=sfix(16)  OutScaling=2^0
  Clock : Clock
      settings: Decimation=10
  Memory : Memory
  Relational Operator : RelationalOperator  Operator=>  LogicOutDataTypeMode=Specify via dialog
  Switch : Switch  Criteria=u2 > Threshold
  Increase : Outport  OutDataType=sfix(16)  OutScaling=2^0
  wires:
  Switch/1 -> Relational Operator/2
  Memory/1 -> Switch/1
  Clock/1 -> Switch/2
  Relational Operator/1 -> Increase/1
  Signal/1 -> Switch/3, Memory/1, Relational Operator/1

== system MIL_Test/Validation Function/Feature extraction/Complete step detection/Step detection/Detect increase2 ==
  Signal : Inport  OutDataType=sfix(16)  OutScaling=2^0
  Clock : Clock
      settings: Decimation=10
  Memory : Memory
  Relational Operator : RelationalOperator  Operator=>  LogicOutDataTypeMode=Specify via dialog
  Switch : Switch  Criteria=u2 > Threshold
  Increase : Outport  OutDataType=sfix(16)  OutScaling=2^0
  wires:
  Signal/1 -> Relational Operator/1, Memory/1, Switch/3
  Relational Operator/1 -> Increase/1
  Clock/1 -> Switch/2
  Memory/1 -> Switch/1
  Switch/1 -> Relational Operator/2

== system MIL_Test/Validation Function/Feature extraction/Complete step detection/Step detection/Hold1 ==
  " " : Inport  OutDataType=sfix(16)  OutScaling=2^0
  "    " : Inport  Port=2  OutDataType=sfix(16)  OutScaling=2^0
  Memory : Memory  Orientation=left
  Switch : Switch  Criteria=u2 ~= 0
  "  " : Outport  OutDataType=sfix(16)  OutScaling=2^0
  wires:
  " "/1 -> Switch/2
  "    "/1 -> Switch/1
  Switch/1 -> "  "/1, Memory/1
  Memory/1 -> Switch/3

== system MIL_Test/Validation Function/Feature extraction/Complete step detection/Step detection reset/Active if signals constant for some specified time ==
  Signal1 : Inport  OutDataType=sfix(16)  OutScaling=2^0
  Signal 2 : Inport  Port=2  OutDataType=sfix(16)  OutScaling=2^0
  Logical Operator1 : Logic  AllPortsSameDT=off  OutDataTypeMode=boolean
  Min Time : Constant  Value=10  OutDataType=sfix(16)  OutScaling=2^0
  MinMax : MinMax  Inputs=2  OutDataType=sfix(16)  OutScaling=2^0
  Relational Operator2 : RelationalOperator  Operator=<=  LogicOutDataTypeMode=boolean
  Switch : Switch  Criteria=u2 ~= 0
  Time since signal constant : Subsystem  TreatAsAtomicUnit=on  mask(Feature extraction block){RT=0.0001}
      mask prompts: RT "Relative tolerance in %"
      mask help: Detect if the signal value is constant (using the last two signal values) allowing for a user-defined relative deviation
      mask CallbackString:
      | if or( (str2double(get_param(gcb,'RT')) < 0), (str2double(get_param(gcb,'RT')) > 100))
      |     error(['Relative tolerance value (' get_param(gcb,'RT') ') out of range. Please give a value between 0 and 100.']);
      | else
      |     set_param([gcb '/Detect constant/Relative tolerance/Relative Tolerance'],'Value',get_param(gcb,'RT'));
      |     set_param([gcb '/Detect constant'],'RT',get_param(gcb,'RT'));
      | end
  Time since signal constant1 : Subsystem  TreatAsAtomicUnit=on  mask(Feature extraction block){RT=0.0001}
      mask prompts: RT "Relative tolerance in %"
      mask help: Detect if the signal value is constant (using the last two signal values) allowing for a user-defined relative deviation
      mask CallbackString:
      | if or( (str2double(get_param(gcb,'RT')) < 0), (str2double(get_param(gcb,'RT')) > 100))
      |     error(['Relative tolerance value (' get_param(gcb,'RT') ') out of range. Please give a value between 0 and 100.']);
      | else
      |     set_param([gcb '/Detect constant/Relative tolerance/Relative Tolerance'],'Value',get_param(gcb,'RT'));
      |     set_param([gcb '/Detect constant'],'RT',get_param(gcb,'RT'));
      | end
  Zero : Constant  Value=0  OutDataType=sfix(16)  OutScaling=2^0
  Constant signals : Outport  OutDataType=sfix(16)  OutScaling=2^0
  wires:
  Zero/1 -> Switch/3
  Logical Operator1/1 -> Switch/2
  MinMax/1 -> Switch/1
  Time since signal constant1/1(Trigger) -> Logical Operator1/2
  Time since signal constant/1(Trigger) -> Logical Operator1/1
  Time since signal constant/2(Feature) -> MinMax/1
  Time since signal constant1/2(Feature) -> MinMax/2
  Switch/1 -> Relational Operator2/2
  Min Time/1 -> Relational Operator2/1
  Relational Operator2/1 -> Constant signals/1
  Signal 2/1 -> Time since signal constant1/1(Signal)
  Signal1/1 -> Time since signal constant/1(Signal)

== system MIL_Test/Validation Function/Feature extraction/Complete step detection/Step detection reset/Step detection ==
  Signal : Inport  OutDataType=sfix(16)  OutScaling=2^0
  Abs : Abs
  Add : Sum  Inputs=+-  OutDataType=sfix(16)  OutScaling=2^-10
  Clock : Clock
      settings: Decimation=10
  Memory : Memory
  Min step size : Constant  Value=10  OutDataType=sfix(16)  OutScaling=2^0
  Relational Operator : RelationalOperator  LogicOutDataTypeMode=boolean
  Switch : Switch  Criteria=u2 > Threshold
  Step : Outport  OutDataType=sfix(16)  OutScaling=2^0
  wires:
  Switch/1 -> Add/2
  Memory/1 -> Switch/1
  Clock/1 -> Switch/2
  Signal/1 -> Add/1, Switch/3, Memory/1
  Abs/1 -> Relational Operator/1
  Min step size/1 -> Relational Operator/2
  Relational Operator/1 -> Step/1
  Add/1 -> Abs/1

== system MIL_Test/Validation Function/Feature extraction/Step response characteristics/Step response characteristics extraction/Expected set point and step parameters ==
  Step/z : Inport  OutDataType=sfix(16)  OutScaling=2^0
  Step : Inport  Port=2  OutDataType=sfix(16)  OutScaling=2^0
  Static Gain : Inport  Port=3  OutDataType=sfix(16)  OutScaling=2^0
  Trigger : TriggerPort
  Compare To Zero : simulink/Logic and Bit Operations/Compare To Zero  SystemSampleTime=-1  relop=>  LogicOutDataTypeMode=uint8  ZeroCross=off
  Divide : Product  Inputs=**  OutDataType=sfix(16)  OutScaling=2^-10
  Divide1 : Product  Inputs=**  OutDataType=sfix(16)  OutScaling=2^-10
  Subtract : Sum  Inputs=-+  OutDataType=sfix(16)  OutScaling=2^-10
  Step sign : Outport  OutDataType=sfix(16)  OutScaling=2^0
  Set point : Outport  Port=2  OutDataType=sfix(16)  OutScaling=2^0
  Response step size : Outport  Port=3  OutDataType=sfix(16)  OutScaling=2^0
  wires:
  Divide1/1 -> Response step size/1
  Compare To Zero/1 -> Step sign/1
  Subtract/1 -> Divide1/1, Compare To Zero/1
  Step/z/1 -> Subtract/1
  Step/1 -> Subtract/2, Divide/1
  Static Gain/1 -> Divide1/2, Divide/2
  Divide/1 -> Set point/1

== system MIL_Test/Validation Function/Feature extraction/Step response characteristics/Step response characteristics extraction/Extract maximum overshoot ==
  Step response : Inport  OutDataType=sfix(16)  OutScaling=2^0
  Reset : Inport  Port=2  OutDataType=sfix(16)  OutScaling=2^0
  Step sign : Inport  Port=3  OutDataType=sfix(16)  OutScaling=2^0
  Active if signals constant for some specified time : Subsystem
  Detect increase : Subsystem  TreatAsAtomicUnit=on
  Detect increase1 : Subsystem  TreatAsAtomicUnit=on
  Detect increase2 : Subsystem  TreatAsAtomicUnit=on
  Hold value with counter : Subsystem  TreatAsAtomicUnit=on
  Logical Operator : Logic  Operator=OR  Inputs=3  AllPortsSameDT=off  OutDataTypeMode=boolean
  Step response moving average and initial conditions before step : Subsystem  TreatAsAtomicUnit=on
  Subtract : Sum  Inputs=+-  OutDataType=sfix(16)  OutScaling=2^-10
  Trigger hold value : Subsystem  TreatAsAtomicUnit=on
  Maximum overshoot : Outport  OutDataType=sfix(16)  OutScaling=2^0
  wires:
  Active if signals constant for some specified time/1(Constant signals) -> Detect increase/1(Signal)
  Reset/1 -> Step response moving average and initial conditions before step/1(Reset), Hold value with counter/1(Reset counter), Detect increase2/1(Signal)
  Step sign/1 -> Trigger hold value/2(Step sign)
  Step response/1 -> Step response moving average and initial conditions before step/2(Step response), Active if signals constant for some specified time/1(Signal1), Active if signals constant for some specified time/2(Signal 2), Subtract/2, Hold value with counter/2(Value)
  Step response moving average and initial conditions before step/1(d(Step Response) average) -> Trigger hold value/1(d(Step Response) average)
  Subtract/1 -> Maximum overshoot/1
  Hold value with counter/1(Held value) -> Subtract/1
  Logical Operator/1 -> Hold value with counter/Trigger
  Detect increase/1(Increase) -> Logical Operator/1
  Detect increase2/1(Increase) -> Logical Operator/2
  Detect increase1/1(Increase) -> Logical Operator/3
  Trigger hold value/1(Overshoot Trigger) -> Detect increase1/1(Signal)

== system MIL_Test/Validation Function/Feature extraction/Step response characteristics/Step response characteristics extraction/Extract rise time ==
  Step response : Inport  OutDataType=sfix(16)  OutScaling=2^0
  Reset : Inport  Port=2  OutDataType=sfix(16)  OutScaling=2^0
  Set point : Inport  Port=3  OutDataType=sfix(16)  OutScaling=2^0
  Response step size : Inport  Port=4  OutDataType=sfix(16)  OutScaling=2^0
  100 % : Constant  Value=100  OutDataType=sfix(16)  OutScaling=2^0
  "100% " : Constant  Value=100  OutDataType=sfix(16)  OutScaling=2^0
  Add1 : Sum  Inputs=-+  OutDataType=sfix(16)  OutScaling=2^-10
  Add2 : Sum  Inputs=+-  OutDataType=sfix(16)  OutScaling=2^-10
  Clock : Clock
      settings: Decimation=10
  Divide : Product  Inputs=**/  OutDataType=sfix(16)  OutScaling=2^-10
  Divide1 : Product  Inputs=**/  OutDataType=sfix(16)  OutScaling=2^-10
  Logical Operator : Logic  Operator=XOR  AllPortsSameDT=off  OutDataTypeMode=boolean
  Logical Operator1 : Logic  Operator=OR  AllPortsSameDT=off  OutDataTypeMode=boolean
  Relational Operator : RelationalOperator  LogicOutDataTypeMode=boolean
  Relational Operator2 : RelationalOperator  Operator=<=  LogicOutDataTypeMode=boolean
  Time difference : Subsystem  TreatAsAtomicUnit=on
  lowerLim : Constant  Value=10  OutDataType=sfix(16)  OutScaling=2^0
  upperLim : Constant  Value=90  OutDataType=sfix(16)  OutScaling=2^0
  Rise time : Outport  OutDataType=sfix(16)  OutScaling=2^0
  wires:
  Add2/1 -> Relational Operator2/2
  Response step size/1 -> Divide1/2, Divide/2
  Set point/1 -> Add2/1, Add1/2
  Add1/1 -> Relational Operator/1
  Divide/1 -> Add1/1
  100 %/1 -> Divide1/3
  "100% "/1 -> Divide/3
  Relational Operator/1 -> Logical Operator/1
  Relational Operator2/1 -> Logical Operator/2
  Divide1/1 -> Add2/2
  upperLim/1 -> Divide1/1
  lowerLim/1 -> Divide/1
  Logical Operator1/1 -> Time difference/Trigger
  Logical Operator/1 -> Logical Operator1/2
  Reset/1 -> Time difference/1(Reset counter), Logical Operator1/1
  Time difference/1(Time difference) -> Rise time/1
  Step response/1 -> Relational Operator2/1, Relational Operator/2
  Clock/1 -> Time difference/2(Clock)

== system MIL_Test/Validation Function/Feature extraction/Step response characteristics/Step response characteristics extraction/Extract settling time ==
  Step response : Inport  OutDataType=sfix(16)  OutScaling=2^0
  Set point : Inport  Port=2  OutDataType=sfix(16)  OutScaling=2^0
  Reset : Inport  Port=3  OutDataType=sfix(16)  OutScaling=2^0
  Step time : Inport  Port=4  OutDataType=sfix(16)  OutScaling=2^0
  " 100%" : Constant  Value=100  OutDataType=sfix(16)  OutScaling=2^0
  Abs : Abs
  Abs1 : Abs
  Add : Sum  Inputs=+-  OutDataType=sfix(16)  OutScaling=2^-10
  Add3 : Sum  Inputs=+-  OutDataType=sfix(16)  OutScaling=2^-10
  Clock1 : Clock
      settings: Decimation=10
  Divide2 : Product  Inputs=**/  OutDataType=sfix(16)  OutScaling=2^-10
  Logical Operator : Logic  Operator=OR  AllPortsSameDT=off  OutDataTypeMode=boolean
  Logical Operator1 : Logic  Operator=NOT  AllPortsSameDT=off  OutDataTypeMode=boolean
  Relational Operator3 : RelationalOperator  Operator=>  LogicOutDataTypeMode=boolean
  Set point percent : Constant  Value=5  OutDataType=sfix(16)  OutScaling=2^0
  Time stamp : Subsystem  TreatAsAtomicUnit=on
  Settling time : Outport  OutDataType=sfix(16)  OutScaling=2^0
  wires:
  Time stamp/1(Time) -> Settling time/1
  Step time/1 -> Add/2
  Add/1 -> Time stamp/1(Clock)
  Clock1/1 -> Add/1
  Abs1/1 -> Relational Operator3/2
  Divide2/1 -> Abs1/1
  " 100%"/1 -> Divide2/3
  Abs/1 -> Relational Operator3/1
  Add3/1 -> Abs/1
  Set point percent/1 -> Divide2/2
  Step response/1 -> Add3/1
  Set point/1 -> Divide2/1, Add3/2
  Relational Operator3/1 -> Logical Operator1/1
  Logical Operator1/1 -> Logical Operator/2
  Reset/1 -> Logical Operator/1
  Logical Operator/1 -> Time stamp/Trigger

== system MIL_Test/Validation Function/Feature extraction/Step response characteristics/Step response characteristics extraction/Extract steady state error ==
  Step response : Inport  OutDataType=sfix(16)  OutScaling=2^0
  Set point : Inport  Port=2  OutDataType=sfix(16)  OutScaling=2^0
  Subtract : Sum  Inputs=+-  OutDataType=sfix(16)  OutScaling=2^-10
  Weighted Moving Average : S-Function  FunctionName=sfix_fir  Parameters=(getdatatypespecs(OutDataType,OutScaling,DblOver,0)),[DoSatur RndMeth-1],DblOver,dolog,mgainval,(getdatatypespecs(GainDataType,GainScaling,DblOver,RadixGroup)),samptime,vinit,OutputDataTypeScalingMode,GainDataTypeScalingMode  mask(Weighted Moving Average){mgainval=ones(1,10), vinit=0.0, samptime=-1, GainDataTypeScalingMode=Inherit via internal rule, GainDataType=sfix( 16 ), MatRadixGroup=Best Precision: Matrix-wise, GainScaling=2^-10, OutputDataTypeScalingMode=Inherit via internal rule, OutDataType=sfix(16), OutScaling=2^-10, LockScale=off, RndMeth=Floor, DoSatur=off}
      mask prompts: mgainval "Weights:"; vinit "Initial condition:"; samptime "Sample time:"; GainDataTypeScalingMode "Gain data type and scaling:"; GainDataType "Parameter data type:     ex. sfix(16),  uint(8), float('single')"; MatRadixGroup "Parameter scaling mode:"; GainScaling "Parameter scaling:    Slope    ex.  2^-9"; OutputDataTypeScalingMode "Output data type and scaling:"; OutDataType "Output data type:     ex.  sfix(16),  uint(8),  float('single')"; OutScaling "Output scaling:    Slope or [Slope Bias]    ex.  2^-9"; LockScale "Lock output scaling so autoscaling tool can't change it"; RndMeth "Round toward:"; DoSatur "Saturate to max or min when overflows occur"
      mask help: Output the weighted moving average of the input.
      mask init:
      | DblOver = 0;
      | dolog = 0;
      | 
      | if MatRadixGroup == 5
      |     RadixGroup = 1; % BEST_PREC_MAT
      | elseif MatRadixGroup == 4
      |     RadixGroup = 2; % BEST_PREC_COL
      | elseif MatRadixGroup == 3
      |     RadixGroup = 3; % BEST_PREC_ROW
      | elseif MatRadixGroup == 2
      |     RadixGroup = 4; % BEST_PREC_ELE
      | else
      |     RadixGroup = 0; % BEST_PREC_OFF
      | end
      mask StyleString: edit,edit,edit,popup(Specify via dialog|Inherit via internal rule),edit,popup(Use Specified Scaling|Best Precision: Element-wise|Best Precision: Row-wise|Best Precision: Column-wise|Best Precision: Matrix-wise),edit,popup(Specify via dialog|Inherit via internal rule|Inherit via back propagation),edit,edit,checkbox,popup(Zero|Nearest|Ceiling|Floor),checkbox
      mask CallbackString: |||fixptdialog(gcbh)|fixptdialog(gcbh)|fixptdialog(gcbh)||fixptdialog(gcbh)|fixptdialog(gcbh)||||
      mask TabNameString: Main,Main,Main,Parameter data types,Parameter data types,Parameter data types,Parameter data types,Signal data types,Signal data types,Signal data types,Signal data types,Signal data types,Signal data types
      mask Display:
      | fprintf(fixpt_fir_mask_data(mgainval,'dispstr'))
      | plot(fixpt_fir_mask_data(mgainval,1),fixpt_fir_mask_data(mgainval,0))
  ss error : Outport  OutDataType=sfix(16)  OutScaling=2^0
  wires:
  Weighted Moving Average/1 -> ss error/1
  Subtract/1 -> Weighted Moving Average/1
  Set point/1 -> Subtract/2
  Step response/1 -> Subtract/1

== system MIL_Test/Validation Function/Feature extraction/Step response characteristics/Step response characteristics extraction/Step time ==
  Clock : Inport  OutDataType=sfix(16)  OutScaling=2^0
  Trigger : TriggerPort
  Time : Outport  OutDataType=sfix(16)  OutScaling=2^0
  wires:
  Clock/1 -> Time/1
